simulink model "BaseEngineController_LS_128"  (Simulink 7.7)
settings: Solver=FixedStepDiscrete  StartTime=0.0  StopTime=10.0  RelTol=1e-3
PreLoadFcn:
  | try, eval([bdroot '_setup']); catch, eval('model_setup', ''); end
InitFcn:
  | try, eval([bdroot '_setup']); catch, eval('model_setup', ''); end
undefined symbols (not defined in the file): ECU565, High, motohawk_build_version, motohawk_trunc_name, motohawk_vardec_config_group, motohawk_vardec_path, True
libraries: MotoHawk_lib x1418, motohawk_control_primitives_lib x183, motohawk_engine_lib x32, simulink x21, motohawk_annotations_lib x9, AutoDoc_lib x8, simulink_extras x4, motohawk_ccp_examples_lib x1, motohawk_control_primitives_motoshare_lib x1
(part 2 of 27)

== system BaseEngineController_LS_128/Foreground/Control/ActuatorCharacterization ==
  Control : Inport
  Sensors : Inport  Port=2
  Diagnsotics : Inport  Port=3
  Bus Creator1 : BusCreator  Inputs=8
  Bus Creator3 : BusCreator
  Bus Selector1 : BusSelector  OutputSignals=AirCalcs.Baro,Raw.LinearSensors.MAP_Angular,RawIndexes.SysVolt09Idx,Raw.RPM,Raw.LinearSensors.FuelPres
  Bus Selector3 : BusSelector  OutputSignals=RawProcessed.TPS
  Bus Selector4 : BusSelector  OutputSignals=Throttle
  Bus Selector5 : BusSelector  OutputSignals=SparkAdv,SparkEnergy,FPC
  CompareTo : motohawk_control_primitives_lib/CompareTo  SystemSampleTime=-1  op===  val=0
  Electronic Throttle Controller : Subsystem  TreatAsAtomicUnit=on
      mask Display:
      | patch([0 0 1 1], [0 0.075 0.075 0], [230/255 0/255 0/255])
      | patch([0 0 1 1], [0.025 0.05 0.05 0.025], [150/255 0/255 0/255])
      | patch([0 0 1 1], [0 0.025 0.025 0], [0/255 0/255 0/255])
      | 
      | disp('Electronic Throttle');
  Injector Characterization : Subsystem  Description=|
      | /* Name: InjGain Unit:ms/mg ClassID:VAR StorageID:FLASH Access:RW4+RW3+NA2+NA1 TypeID:UINT2 Gain:0.0001       
      |    Min:0.0000 Max:6.5500 Format:5.4 UpdateID:REMOTE Group:"Actuators | Injectors | Config" Help:"Gain valued "
      |    "used in the linear transformation of FPC to mechanical pulsewidth." VardecSig:6C */                       
      |                                                                                                               
      | /* Name: InjOfst Unit:ms ClassID:VAR StorageID:FLASH Access:RW4+RW3+NA2+NA1 TypeID:SINT2 Gain:0.0001          
      |    Min:-3.2768 Max:3.2767 Format:5.4 UpdateID:REMOTE Group:"Actuators | Injectors | Config" Help:"Offset "    
      |    "valued used in the linear transformation of FPC to mechanical pulsewidth." VardecSig:6C */                
      |                                                                                                               
      | /* Name: SysVolt10IdxArr Unit:volt ClassID:ORDARR StorageID:FLASH Access:RW4+RW3+NA2+NA1 TypeID:UINT1         
      |    Gain:0.1 Min:0.00 Max:25.50 Format:4.2 UpdateID:REMOTE OrdLen:10 Group:"Global Index Arrays | Voltage"     
      |    Help:"Ten breakpoint system voltage index array." VardecSig:6C */                                          
      |                                                                                                               
      | /* Name: InjTurnOnTbl Unit:ms ClassID:TBL StorageID:FLASH Access:RW4+RW3+NA2+NA1 TypeID:UINT2 Gain:0.001      
      |    Min:0.0000 Max:65.5350 Format:5.4 UpdateID:REMOTE OrdArr:SysVolt10IdxArr Group:"Actuators | Injectors"     
      |    Help:"Injector turn on time as a function of system voltage." VardecSig:6C */                              
      |                                                                                                               
      | /* Name: InjDeltaPress10IdxArr Unit:kPa ClassID:ORDARR StorageID:FLASH Access:RW4+RW3+NA2+NA1 TypeID:UINT2    
      |    Gain:0.1 Min:0.0 Max:6553.0 Format:5.1 UpdateID:REMOTE OrdLen:10 Group:"Actuators | Injectors" Help:"Ten " 
      |    "breakpoint fuel delta pressure index array." VardecSig:6C */                                              
      |                                                                                                               
      | /* Name: FueldPCompTbl Unit:kPa ClassID:TBL StorageID:FLASH Access:RW4+RW3+NA2+NA1 TypeID:UINT2 Gain:0.1      
      |    Min:0.0 Max:6553.0 Format:5.1 UpdateID:REMOTE OrdArr:InjDeltaPress10IdxArr Group:"Actuators | Injectors"   
      |    Help:"Injector delta pressure compensation table." VardecSig:6C */                                         
      |                                                                                                               
      | /* Name: InjTurnOffTbl Unit:ms ClassID:TBL StorageID:FLASH Access:RW4+RW3+NA2+NA1 TypeID:UINT2                
      |    Gain:0.01 Min:0.00 Max:655.00 Format:5.2 UpdateID:REMOTE OrdArr:InjDeltaPress10IdxArr Group:"Actuators | " 
      |    "Injectors" Help:"Injector turn off time table." VardecSig:6C */                                           
      |                                                                                                               
      | /* Name: InjMPW Unit:ms ClassID:VAR StorageID:RAM Access:RO4+RO3+NA2+NA1 TypeID:UINT2 Gain:0.01 Min:0.00      
      |    Max:655.35 Format:5.2 UpdateID:BACKGND Group:"Actuators | Injectors" Help:"Injector mechanical pulse "     
      |    "width." VardecSig:6C */                                                                                   
      |                                                                                                               
      | /* Name: InjEPW Unit:ms ClassID:VAR StorageID:RAM Access:RO4+RO3+NA2+NA1 TypeID:UINT2 Gain:0.01 Min:0.00      
      |    Max:655.35 Format:5.2 UpdateID:BACKGND Group:"Actuators | Injectors" Help:"Injector electrical pulse "     
      |    "width." VardecSig:6C */                                                                                   
      |                                                                                                               
      | /* Name: InjDeltaPress Unit:kPa ClassID:VAR StorageID:RAM Access:RO4+RO3+NA2+NA1 TypeID:UINT2 Gain:0.01       
      |    Min:0.00 Max:655.35 Format:5.2 UpdateID:BACKGND Group:"Actuators | Injectors" Help:"Delta pressure across "
      |    "the injector." VardecSig:6C */                                                                            
      | /* Name: FuelFlowCompMap Unit:mult ClassID:MAP StorageID:RAM Access:RO4+RO3+NA2+NA1 TypeID:UINT2              
      |    Gain:0.0001 Min:0.0000 Max:2.0000 Format:5.4 UpdateID:BACKGND XOrdArr:IndTorque10IdxArr YOrdArr:RPM10IdxArr
      |    Group:"Actuators | Injectors" Help:"Correction for injector fuel flow differences between injector test "  
      |    "bench and engine operating in the conditions. This map should only be calibrated after volumetric "       
      |    "efficiency has been calibrated to a reference airflow measurement device." VardecSig:6C */
      mask Description: Injector characterization block.
      mask Help: Converts the calculated fuel charge mass (FPC) value to the required electrical pulsewidth. Requires gain, offset, turn-on time vs. voltage, turn-off time vs. injector delta pressure and delta pressure pulsewidth compensation. A choice of five different injector delta pressure calculation methods are offered.
      mask Display:
      | patch([0 0 1 1], [0 0.075 0.075 0], [230/255 0/255 0/255])
      | patch([0 0 1 1], [0.025 0.05 0.05 0.025], [150/255 0/255 0/255])
      | patch([0 0 1 1], [0 0.025 0.025 0], [0/255 0/255 0/255])
      | 
      | disp('INJECTOR\nCHRZN.\n(High Z Only)')
  SequenceCutPattern : Subsystem
      mask Display:
      | patch([0 0 1 1], [0 0.075 0.075 0], [230/255 0/255 0/255])
      | patch([0 0 1 1], [0.025 0.05 0.05 0.025], [150/255 0/255 0/255])
      | patch([0 0 1 1], [0 0.025 0.025 0], [0/255 0/255 0/255])
      | 
      | disp('REV LIMITER\nACTION\n8 CYLINDER')
  Spark Advance to Start Angle : Subsystem  Description=|  TreatAsAtomicUnit=on
      | /* Name: CoilDrvrDlyTime Unit:us ClassID:VAR StorageID:FLASH Access:RW4+RW3+NA2+NA1 TypeID:UINT2 Gain:0.1       
      |    Min:0.00 Max:6553.50 Format:6.2 UpdateID:REMOTE Group:"Actuators | Coils" Help:"Coil driver delay time "     
      |    "between initiation of the EST signal and the initiation of coil dwell." VardecSig:6C */                     
      |                                                                                                                 
      | /* Name: SysVolt10IdxArr Unit:volt ClassID:VAR StorageID:FLASH Access:RW4+RW3+NA2+NA1 TypeID:UINT1 Gain:0.1     
      |    Min:0.00 Max:25.50 Format:4.2 UpdateID:REMOTE Group:"Global Index Arrays | Voltage" Help:"Ten breakpoint "   
      |    "system voltage index array." VardecSig:6C */                                                                
      |                                                                                                                 
      | /* Name: SpkEnergy10IdxArr Unit:volt ClassID:VAR StorageID:FLASH Access:RW4+RW3+NA2+NA1 TypeID:UINT1            
      |    Gain:0.1 Min:0.00 Max:25.50 Format:4.2 UpdateID:REMOTE Group:"Actuators | Coils" Help:"Ten breakpoint spark "
      |    "energy index array." VardecSig:6C */                                                                        
      |                                                                                                                 
      | /* Name: CoilDwellMap Unit:ms ClassID:MAP StorageID:FLASH Access:RW4+RW3+NA2+NA1 TypeID:UINT2 Gain:0.01         
      |    Min:0.00 Max:655.35 Format:4.2 UpdateID:REMOTE XOrdArr:SpkEnergy10IdxArr YOrdArr:SysVolt10IdxArr             
      |    Group:"Actuators | Coils" Help:"Required coil dwell map as a function of system voltage and spark energy."   
      |    VardecSig:6C */
      mask Type: Stop Angle to Start Angle
      mask Description: Stop Angle to Start Angle calculation.  Subtracts the duration of a Pulse Width in the angle domain from a given Stop Angle.
      mask Display:
      | patch([0 0 1 1], [0 0.075 0.075 0], [230/255 0/255 0/255])
      | patch([0 0 1 1], [0.025 0.05 0.05 0.025], [150/255 0/255 0/255])
      | patch([0 0 1 1], [0 0.025 0.025 0], [0/255 0/255 0/255])
  Spark Coil Characterization : Subsystem  Description=|  TreatAsAtomicUnit=on
      | /* Name: CoilDrvrDlyTime Unit:us ClassID:VAR StorageID:FLASH Access:RW4+RW3+NA2+NA1 TypeID:UINT2 Gain:0.1       
      |    Min:0.00 Max:6553.50 Format:6.2 UpdateID:REMOTE Group:"Actuators | Coils" Help:"Coil driver delay time "     
      |    "between initiation of the EST signal and the initiation of coil dwell." VardecSig:6C */                     
      |                                                                                                                 
      | /* Name: SysVolt10IdxArr Unit:volt ClassID:VAR StorageID:FLASH Access:RW4+RW3+NA2+NA1 TypeID:UINT1 Gain:0.1     
      |    Min:0.00 Max:25.50 Format:4.2 UpdateID:REMOTE Group:"Global Index Arrays | Voltage" Help:"Ten breakpoint "   
      |    "system voltage index array." VardecSig:6C */                                                                
      |                                                                                                                 
      | /* Name: SpkEnergy10IdxArr Unit:volt ClassID:VAR StorageID:FLASH Access:RW4+RW3+NA2+NA1 TypeID:UINT1            
      |    Gain:0.1 Min:0.00 Max:25.50 Format:4.2 UpdateID:REMOTE Group:"Actuators | Coils" Help:"Ten breakpoint spark "
      |    "energy index array." VardecSig:6C */                                                                        
      |                                                                                                                 
      | /* Name: CoilDwellMap Unit:ms ClassID:MAP StorageID:FLASH Access:RW4+RW3+NA2+NA1 TypeID:UINT2 Gain:0.01         
      |    Min:0.00 Max:655.35 Format:4.2 UpdateID:REMOTE XOrdArr:SpkEnergy10IdxArr YOrdArr:SysVolt10IdxArr             
      |    Group:"Actuators | Coils" Help:"Required coil dwell map as a function of system voltage and spark energy."   
      |    VardecSig:6C */
      mask Description: Coil characterization block.
      mask Help: Given the desired spark energy and system voltage, this block determines the required coil dwell period. Requires calibration of the dwell map and the delay time.
      mask Display:
      | patch([0 0 1 1], [0 0.075 0.075 0], [230/255 0/255 0/255])
      | patch([0 0 1 1], [0.025 0.05 0.05 0.025], [150/255 0/255 0/255])
      | patch([0 0 1 1], [0 0.025 0.025 0], [0/255 0/255 0/255])
      | 
      | disp('COIL\nCHRZN.')
  motohawk_data_read : MotoHawk_lib/Data Storage Blocks/motohawk_data_read  source=Lookup By Name  structure=Scalar  operation=Read scalar from location by index  sz_vec=4  sz_row=2  sz_col=3  typ=boolean  nam='AirControlSource'  checkNull=on  struct_inst_name='Struct1'  struct_nam='MyStruct'
  motohawk_trigger : MotoHawk_lib/Trigger Blocks/motohawk_trigger  Tag=Trigger  trigger=FGND_5XRTI_PERIODIC  function_name=Trigger_FGND_5XRTI_PERIODIC_1093p0005  priority_order=1  inherited=on  run_disabled=off  override_app_monitor=off  target=ECU565_128
  motohawk_trigger1 : MotoHawk_lib/Trigger Blocks/motohawk_trigger  Tag=Trigger  trigger=FGND_5XRTI_PERIODIC  function_name=Trigger_FGND_5XRTI_PERIODIC_1094p0005  priority_order=1  inherited=on  run_disabled=off  override_app_monitor=off  target=ECU565_128
  Actuators : Outport
  wires:
  Sensors/1 -> Bus Selector1/1, Bus Creator3/3, Bus Selector3/1  "Sensors"
  Bus Selector3/1 -> Electronic Throttle Controller/1(TPS)  "<TPS>"
  Electronic Throttle Controller/1(ETC) -> Bus Creator1/5  "ETC"
  Bus Selector4/1 -> Electronic Throttle Controller/2(ETCReq)  "<Throttle>"
  Control/1 -> Bus Selector5/1, Bus Creator3/2, Bus Selector4/1  "Controller"
  Bus Selector1/3 -> Injector Characterization/4(SysVolt09Idx), Spark Coil Characterization/2(SysVolt09Idx)  "<SysVolt09Idx>"
  Bus Selector1/4 -> Spark Advance to Start Angle/2(RPM), Injector Characterization/5(RPM)  "<RPM>"
  Spark Advance to Start Angle/1(Start Angle [degCA]) -> Bus Creator1/3  "SparkStartAngle"
  Spark Coil Characterization/1(SparkDwell [ms]) -> Spark Advance to Start Angle/3(PulseWidth [ms])  "SparkDwell"
  Bus Selector1/2 -> Injector Characterization/3(MAP [kPa])  "<MAP_Angular>"
  Bus Selector1/1 -> Injector Characterization/2(BaroPress [kPa])  "<Baro>"
  Injector Characterization/1(MPW [ms]) -> Bus Creator1/1  "InjMPW"
  Bus Selector5/1 -> Spark Advance to Start Angle/1(Stop Angle [degCA])  "<SparkAdv>"
  Bus Selector5/2 -> Spark Coil Characterization/1(SparkEnergy [mJ])  "<SparkEnergy>"
  Spark Coil Characterization/2(SparkEnable [bool]) -> Bus Creator1/4  "SparkEnable"
  Injector Characterization/2(EPWOffset [ms]) -> Bus Creator1/2  "InjEPWOffset"
  SequenceCutPattern/1(Spark) -> Bus Creator1/6  "SparkCutSeq"
  SequenceCutPattern/2(Fuel) -> Bus Creator1/7  "FuelCutSeq"
  Bus Creator3/1 -> Actuators/1  "Engine"
  Bus Creator1/1 -> Bus Creator3/4  "ActuatorCharacterization"
  Diagnsotics/1 -> Bus Creator3/1  "Diagnsotics"
  motohawk_trigger/1 -> Spark Advance to Start Angle/Trigger
  motohawk_trigger1/1 -> Spark Coil Characterization/Trigger
  motohawk_data_read/1 -> CompareTo/1
  CompareTo/1 -> Electronic Throttle Controller/Enable
  Electronic Throttle Controller/2(ETC_TestActive) -> Bus Creator1/8  "ETC_TestActive"
  Bus Selector1/5 -> Injector Characterization/6(FuelPress [kPa])  "<FuelPres>"
  Bus Selector5/3 -> Injector Characterization/1(FPC [mg])  "<FPC>"

== system BaseEngineController_LS_128/Foreground/Control/Controller ==
  Sensors : Inport
  Bus Selector : BusSelector  OutputSignals=RawProcessed.EngineState
  Crank : Subsystem  TreatAsAtomicUnit=on
      mask Display: disp('CRANK STATE\nALGORITHM');
  Crank State : motohawk_control_primitives_lib/CompareTo  SystemSampleTime=-1  op===  val=2
  Merge : Subsystem
  Run : Subsystem  TreatAsAtomicUnit=on
      mask Display: disp('RUN STATE\nALGORITHM');
  Run State : motohawk_control_primitives_lib/CompareTo  SystemSampleTime=-1  op===  val=3
  Stall : Subsystem  TreatAsAtomicUnit=on
      mask Display: disp('STALL STATE\nALGORITHM');
  Stall State : motohawk_control_primitives_lib/CompareTo  SystemSampleTime=-1  op===  val=1
  Actuators : Outport
  DesEquivRatio : Outport  Port=2
  wires:
  Sensors/1 -> Bus Selector/1, Crank/1(Inputs), Run/1(Inputs), Stall/1(Inputs)
  Stall State/1 -> Stall/Enable
  Crank State/1 -> Crank/Enable
  Run State/1 -> Run/Enable
  Stall/1(Actuators) -> Merge/1(Stall)
  Run/1(Actuators) -> Merge/3(Run)
  Crank/1(Actuators) -> Merge/2(Crank)
  Bus Selector/1 -> Stall State/1, Run State/1, Crank State/1  "<EngineState>"
  Merge/1(Actuators) -> Actuators/1
  Run/2(DesEquivRatio) -> DesEquivRatio/1

== system BaseEngineController_LS_128/Foreground/Control/Diagnostics ==
  Control : Inport
  Sensors : Inport  Port=2
  DesEquivRatio : Inport  Port=3
  Trigger : TriggerPort  TriggerType=function-call
  AC Fault : Subsystem
  AirFlow : Subsystem
  Boost Fault : Subsystem
  Bus Creator1 : BusCreator
  Bus Selector : BusSelector  OutputSignals=Raw.RPMInst
  Digital Sensors : Subsystem
  Engine Overheat Fault Logic : Subsystem
  Fuel Economy : Subsystem
  Lean Protect : Subsystem
  Low Oil Pressure Fault Logic : Subsystem
  Low Voltage : Subsystem
  MAP Fault Logic : Subsystem
  MISFIRE : Subsystem
  O2 Smart Sensor : Subsystem
  Overspeed Protection : Subsystem  AncestorBlock=motohawk_engine_lib/Overspeed Protection
      mask Description:
      | Block allows for three levels of overspeed rev limits, and will set three fault accordingly.
      | 
      | Soft Overspeed, Medium Overspeed, and Hard Overspeed.
      mask Display:
      | patch([0 0 1 1], 0.5*[0 0.075 0.075 0], [230/255 0/255 0/255])
      | patch([0 0 1 1], 0.5*[0.025 0.05 0.05 0.025], [150/255 0/255 0/255])
      | patch([0 0 1 1], 0.5*[0 0.025 0.025 0], [0/255 0/255 0/255])
      | 
      | disp('RPM LIMITER');
  Terminator2 : Terminator
  Wrong Fuel Pressure Fault Logic : Subsystem
  Diagnostics : Outport
  wires:
  Bus Creator1/1 -> Diagnostics/1  "Diagnostics"
  Sensors/1 -> Bus Selector/1, Engine Overheat Fault Logic/1(Sensors), MAP Fault Logic/1(Sensors), Low Oil Pressure Fault Logic/1(Sensors), Fuel Economy/1(Sensors), Wrong Fuel Pressure Fault Logic/1(Sensors), Boost Fault/1(Sensors), AC Fault/1(Sensors), Lean Protect/1(Sensors), Low Voltage/1(Sensors), Digital Sensors/1(Sensors), O2 Smart Sensor/1(Sensors), MISFIRE/1(Sensors), AirFlow/1(Sensors)
  Control/1 -> Terminator2/1, Fuel Economy/2(Controller), Boost Fault/2(Controller), AC Fault/2(Controller)  "Control"
  Bus Selector/1 -> Overspeed Protection/1(RPM)  "<RPMInst>"
  Fuel Economy/1(FuelEconomy_instantaneous) -> Bus Creator1/3  "FuelEconomy_instantaneous"
  Fuel Economy/2(FuelEconomy_filtered) -> Bus Creator1/4  "FuelEconomy_filtered"
  Low Oil Pressure Fault Logic/1(LowOilPres) -> Bus Creator1/2  "LowOilPres"
  Engine Overheat Fault Logic/1(Overheat_Warning) -> Bus Creator1/1  "Overheat_Warning"
  DesEquivRatio/1 -> O2 Smart Sensor/2(DesEquivRatio)

== system BaseEngineController_LS_128/Foreground/Control/VirtualSensors ==
  Raw : Inport
  AirCalcs : Subsystem
  Bus Creator : BusCreator  Inputs=7
  FuelLevel : Subsystem
  LoadBasedCalcs : Subsystem
  Raw Indexes : Subsystem
  RawProcessed : Subsystem
  Virtual Indexes : Subsystem
  Sensors : Outport
  wires:
  Raw/1 -> RawProcessed/1(Raw), Raw Indexes/1(Raw), AirCalcs/2(Raw), LoadBasedCalcs/1(RAW), FuelLevel/1(Sensors), Bus Creator/1  "Raw"
  Bus Creator/1 -> Sensors/1  "SynthSensors"
  RawProcessed/1(RawProcessed) -> Bus Creator/2, AirCalcs/4(RawProcessed), Virtual Indexes/2(RawProcessed), FuelLevel/2(Raw Processed), Raw Indexes/2(RawProcessed)  "RawProcessed"
  Raw Indexes/1(RawIndexes) -> Bus Creator/3, AirCalcs/1(RawIndexes), RawProcessed/2(Indexes)  "RawIndexes"
  AirCalcs/1(AirCalcs) -> Bus Creator/4, Virtual Indexes/1(AirCalcs)  "AirCalcs"
  LoadBasedCalcs/1(SSEng) -> Bus Creator/5, AirCalcs/3(SSEngOpr)  "SSEng"
  Virtual Indexes/1(VirtualIndexes) -> Bus Creator/6  "VirtualIndexes"
  FuelLevel/1(Fuel Lvl Final) -> Bus Creator/7  "FuelLvl_Fin"

== system BaseEngineController_LS_128/Foreground/Inputs/CAN ==
  AEM GPS : Subsystem
  AEM X Lambda : Subsystem
  Bus Creator1 : BusCreator
  SensorBus : Outport
  wires:
  Bus Creator1/1 -> SensorBus/1  "CAN"
  AEM X Lambda/1(O2_BankA) -> Bus Creator1/1  "O2_BankA"
  AEM GPS/1(GPS_BUS) -> Bus Creator1/4  "GPS_BUS"
  AEM X Lambda/3(O2_BUS) -> Bus Creator1/3  "O2_BUS"
  AEM X Lambda/2(O2_BankB) -> Bus Creator1/2  "O2_BankB"

== system BaseEngineController_LS_128/Foreground/Inputs/Digital ==
  "ACSw " : motohawk_engine_lib/Analog Switch  SystemSampleTime=-1  nam='ACSw'  prefix='ACSw'  switchpoint=500  polarity=High-True  parent_group=motohawk_vardec_path(gcb)
  Bus Creator : BusCreator  Inputs=6
  ClutchSw : motohawk_engine_lib/Analog Switch  SystemSampleTime=-1  nam='ClutchSw'  prefix='ClutchSw'  switchpoint=500  polarity=High-True  parent_group=motohawk_vardec_path(gcb)
  Data Type Conversion : DataTypeConversion
  Data Type Conversion1 : DataTypeConversion
  ESTOP : motohawk_engine_lib/Analog Switch1  SystemSampleTime=-1  nam='ESTOP'  prefix='ESTOP'  polarity=High-True  parent_group=motohawk_vardec_path(gcb)
  Gain : Gain  Gain=.01
  Gain1 : Gain  Gain=.01
  MAF_Sensor : motohawk_engine_lib/Non-Linear Sensor Characterization (tbl)  SystemSampleTime=-1  nam='MAF'  prefix='MAF'  units='g/s'  inputunits='Hz'  parent_group=motohawk_vardec_path(gcb)  tblsize=13  samp_time=-1
  "Scramble " : Subsystem  AncestorBlock=motohawk_engine_lib/Analog Switch  mask{nam='Scramble', prefix='Scramble', switchpoint=500, polarity=High-True, parent_group=motohawk_vardec_path(gcb)}
      mask prompts: nam "Name"; switchpoint "Switch Point (ADC)"; parent_group "MotoTune Group"
      mask init:
      | lbl = ['Analog Switch: ' nam ' [bool]'];
      | group = [parent_group ' | ' nam];
      mask StyleString: edit,edit,edit,popup(High-True|Low-True),edit
      mask Display:
      | patch([0 0 1 1], [0 0.075 0.075 0], [230/255 0/255 0/255])
      | patch([0 0 1 1], [0.025 0.05 0.05 0.025], [150/255 0/255 0/255])
      | patch([0 0 1 1], [0 0.025 0.025 0], [0/255 0/255 0/255])
      | 
      | disp(lbl);
  Terminator{1..4} (4 alike) : Terminator
  VSPD : motohawk_engine_lib/Non-Linear Sensor Characterization (tbl)  SystemSampleTime=-1  nam='VSPD'  prefix='VSPD'  units='MPH'  inputunits='Hz'  parent_group=motohawk_vardec_path(gcb)  tblsize=5  samp_time=-1
  VSPD_Filt : Subsystem
  motohawk_ain1 : MotoHawk_lib/Analog I//O Blocks/motohawk_ain  res_name=[]  text_resource=AN15M  code_resource=RES_ECUP  val_resource=-1  target=ECU565-128  resource_enum_str=(None)=-1,ECUP=53,DRVP=54,XDRP=55,AN1M=56,AN2M=57,AN3M=58,AN4M=59,AN5M=60,AN6M=61,AN7M=62,AN8M=63,AN9M=64,AN10M=65,AN11M=66,AN12M=67,AN13M=68,AN14M=69,AN15M=70,AN16M=71,AN17M=72,AN18M=73,AN19M=74,AN20M=75,AN21M=76,AN22M=77,AN23M=78,AN24M=79,AN25M=80,AN26M=81,AN27M=82,AN28M=83,AN29M=84,AN30M=85,AN31M=86,AN32M=87,AN33M=88,AN34M=89,O2A=90,O2B=91,XDRP_B=92,REF_14V=143  altref=5V Reference  typ=uint16  num_adc_bits=10  use_stat=off  use_vardec=on  nam='ClutchSw_Pin'  read_level=1  write_level=1  group='System | I/O Pins | Inputs Config'
  motohawk_ain5 : MotoHawk_lib/Analog I//O Blocks/motohawk_ain  res_name=[]  text_resource=AN15M  code_resource=RES_ECUP  val_resource=-1  target=ECU565-128  resource_enum_str=(None)=-1,ECUP=53,DRVP=54,XDRP=55,AN1M=56,AN2M=57,AN3M=58,AN4M=59,AN5M=60,AN6M=61,AN7M=62,AN8M=63,AN9M=64,AN10M=65,AN11M=66,AN12M=67,AN13M=68,AN14M=69,AN15M=70,AN16M=71,AN17M=72,AN18M=73,AN19M=74,AN20M=75,AN21M=76,AN22M=77,AN23M=78,AN24M=79,AN25M=80,AN26M=81,AN27M=82,AN28M=83,AN29M=84,AN30M=85,AN31M=86,AN32M=87,AN33M=88,AN34M=89,O2A=90,O2B=91,XDRP_B=92,REF_14V=143  altref=5V Reference  typ=uint16  num_adc_bits=10  use_stat=off  use_vardec=on  nam='ACSwPin'  read_level=1  write_level=1  group='System | I/O Pins | Inputs Config'
  motohawk_ain6 : MotoHawk_lib/Analog I//O Blocks/motohawk_ain  res_name=[]  text_resource=AN19M  code_resource=RES_ECUP  val_resource=-1  target=ECU565-128  resource_enum_str=(None)=-1,ECUP=53,DRVP=54,XDRP=55,AN1M=56,AN2M=57,AN3M=58,AN4M=59,AN5M=60,AN6M=61,AN7M=62,AN8M=63,AN9M=64,AN10M=65,AN11M=66,AN12M=67,AN13M=68,AN14M=69,AN15M=70,AN16M=71,AN17M=72,AN18M=73,AN19M=74,AN20M=75,AN21M=76,AN22M=77,AN23M=78,AN24M=79,AN25M=80,AN26M=81,AN27M=82,AN28M=83,AN29M=84,AN30M=85,AN31M=86,AN32M=87,AN33M=88,AN34M=89,O2A=90,O2B=91,XDRP_B=92,REF_14V=143  altref=5V Reference  typ=uint16  num_adc_bits=10  use_stat=off  use_vardec=on  nam='ScramblePin'  read_level=1  write_level=1  group='System | I/O Pins | Inputs Config'
  motohawk_callout1 : motohawk_annotations_lib/motohawk_callout1  BlockType_='Mototron_harea'  desc='\fontsize{12}Read from H/W'  edit_text=Compute the mean forward body acceleration.Worry about rounding.  edit_as=255
  motohawk_callout2 : motohawk_annotations_lib/motohawk_callout1  BlockType_='Mototron_harea'  desc='\fontsize{12}Convert to Engineering Units'  edit_text=Compute the mean forward body acceleration.Worry about rounding.  edit_as=255
  motohawk_callout3 : motohawk_annotations_lib/motohawk_callout1  BlockType_='Mototron_harea'  desc='\fontsize{12}Create a Bus of Sensors'  edit_text=Compute the mean forward body acceleration.Worry about rounding.  edit_as=255
  motohawk_din : MotoHawk_lib/Digital I//O Blocks/motohawk_din  resource_name=[]  text_resource=O2A  code_resource=NONE  val_resource=-1  target=ECU565-128  resource_enum_str=(None)=-1,AN1M=56,AN2M=57,AN3M=58,AN4M=59,AN5M=60,AN6M=61,AN7M=62,AN8M=63,AN9M=64,AN10M=65,AN11M=66,AN12M=67,AN13M=68,AN14M=69,AN15M=70,AN16M=71,AN17M=72,AN18M=73,AN19M=74,AN20M=75,AN21M=76,AN22M=77,AN23M=78,AN24M=79,AN25M=80,AN26M=81,AN27M=82,AN28M=83,AN29M=84,AN30M=85,AN31M=86,AN32M=87,AN33M=88,AN34M=89,O2A=90,O2B=91,DG1M=93,DG2M=94,DG3M=95,DG4M=96,DG5M=102,DG6M=103,DG7M=104,SPD1=105,SPD2=106,DG8M=111  pullup=None  use_stat=off  use_vardec=on  nam='ESTOPPin'  read_level=1  write_level=1  group='System | I/O Pins | Inputs Config'
  motohawk_frequency_in1 : MotoHawk_lib/Advanced Digital I//O/motohawk_frequency_in  res_name=[]  text_resource=DG4M  code_resource=RES_DG1M  val_resource=-1  target=ECU565-128  resource_enum_str=(None)=-1,DG1M=93,DG2M=94,DG3M=95,DG4M=96,DG5M=102,DG6M=103,DG7M=104,SPD1=105,SPD2=106,DG8M=111  ipwm=Perform Duty Cycle Measument  itrig=off  Nmax=8  edge=Falling Edge  alias=Disabled  min_freq=10  sig=Digital Input  use_vardec=on  nam='VSPD_Pin'  read_level=1  write_level=1  group='System | I/O Pins | Inputs Config'  cal_group='System | I/O Pins | Frequency In Config'
  motohawk_frequency_in2 : MotoHawk_lib/Advanced Digital I//O/motohawk_frequency_in  res_name=[]  text_resource=DG2M  code_resource=RES_DG1M  val_resource=-1  target=ECU565-128  resource_enum_str=(None)=-1,DG1M=93,DG2M=94,DG3M=95,DG4M=96,DG5M=102,DG6M=103,DG7M=104,SPD1=105,SPD2=106,DG8M=111  ipwm=Perform Duty Cycle Measument  itrig=off  Nmax=8  edge=Falling Edge  alias=Disabled  min_freq=10  sig=Digital Input  use_vardec=on  nam='MAF_Pin'  read_level=1  write_level=1  group='System | I/O Pins | Inputs Config'  cal_group='System | I/O Pins | Frequency In Config'
  SensorBus : Outport
  wires:
  Bus Creator/1 -> SensorBus/1  "Digital"
  motohawk_frequency_in2/1 -> Data Type Conversion/1
  MAF_Sensor/2 -> Terminator4/1
  Data Type Conversion/1 -> Gain/1
  Gain/1 -> MAF_Sensor/1
  motohawk_frequency_in2/2 -> Terminator1/1
  motohawk_ain5/1 -> "ACSw "/1
  motohawk_ain6/1 -> "Scramble "/1(ADC)
  motohawk_din/1 -> ESTOP/1
  MAF_Sensor/1 -> Bus Creator/1  "MAF"
  ESTOP/1 -> Bus Creator/2  "ESTOP"
  motohawk_frequency_in1/1 -> Data Type Conversion1/1
  Data Type Conversion1/1 -> Gain1/1
  Gain1/1 -> VSPD/1
  motohawk_frequency_in1/2 -> Terminator2/1
  VSPD/2 -> Terminator3/1
  motohawk_ain1/1 -> ClutchSw/1
  VSPD/1 -> VSPD_Filt/1(In1)  "VSPD"
  "ACSw "/1 -> Bus Creator/3  "ACSw"
  "Scramble "/1(DiscOut) -> Bus Creator/4  "Scramble"
  VSPD_Filt/1(Out1) -> Bus Creator/5  "VSPD"
  ClutchSw/1 -> Bus Creator/6  "ClutchSw"

== system BaseEngineController_LS_128/Foreground/Inputs/EngineSpeed ==
  note: Set PseudoRPM from MotoTune
      | to a non-zero value to cause
      | simulated RPM
  Constant : Constant  Value=0  OutDataTypeStr=Inherit: Inherit via back propagation
  Data Type Conversion : DataTypeConversion  SaturateOnIntegerOverflow=on  RndMeth=Zero
  Data Type Conversion1 : DataTypeConversion  OutDataTypeStr=double  SaturateOnIntegerOverflow=on  RndMeth=Zero
  Data Type Conversion3 : DataTypeConversion  RndMeth=Zero
  Encoder Diagnostics : Subsystem
  First Order Low Pass (Tunable)1 : motohawk_control_primitives_lib/First Order Low Pass (Tunable)  SystemSampleTime=-1  nam='RPMFiltConst'  samp_time=-1  group=motohawk_vardec_path(gcb)
  Gain : Gain  Gain=16  SaturateOnIntegerOverflow=on  OutDataTypeStr=Inherit: Same as input  ParamDataTypeStr=Inherit: Same as input
  Relational Operator : RelationalOperator  Operator=~=  ZeroCross=off  InputSameDT=on
  motohawk_calibration : MotoHawk_lib/Calibration & Probing Blocks/motohawk_calibration  nam='PseudoRPM'  val=0  storage=Calibration  show_more=on  name_source=Use Parameter  data_type=Inherit via back propagation  read_level=1  write_level=1  ovr_cals=on  view_as=Number  enum_struct={'Disabled', 'Enabled'}  vector_style=Wide Row  use_help_units=off  help=''  units=''  use_header_enum=off  row_header_enum={}  col_header_enum={}  use_min_max=off  min_val=-inf  max_val=inf  use_precision=off  precision=''  gain=1  offset=0  exp=1  use_mototune_group=on  mototune_group=motohawk_vardec_path(gcb)
  motohawk_calibration1 : MotoHawk_lib/Calibration & Probing Blocks/motohawk_calibration  nam='EngineToEncoderOffset'  val=0  storage=Calibration  show_more=on  name_source=Use Parameter  data_type=Inherit from 'Default Value'  read_level=1  write_level=1  ovr_cals=on  view_as=Number  enum_struct={'Disabled', 'Enabled'}  vector_style=Wide Row  use_help_units=on  help=''  units=''  use_header_enum=off  row_header_enum={}  col_header_enum={}  use_min_max=off  min_val=-inf  max_val=inf  use_precision=off  precision=''  gain=1  offset=0  exp=1  use_mototune_group=on  mototune_group=motohawk_vardec_path(gcb)
  motohawk_encoder_average_rpm : MotoHawk_lib/Encoder Blocks/motohawk_encoder_average_rpm
  motohawk_encoder_def : MotoHawk_lib/Encoder Blocks/motohawk_encoder_def  encoder_type=GM 24Xe - 4-Stroke - Half-Moon CAM  interface=Digital Crank - Digital Cam  sync=Rising Edge  crnkpullup=Strong Pullup  camsync=Rising Edge  campullup=Strong Pullup  angle_offset=27  sec_tdcoffset=-34.3  cam_delay=0  teeth_after_cam=-1  ignore_teeth=6  ignore_delay=100  angles=[0 270 630 540 450 360 180 90]  cnk_align_with_cam=off  adaptive_vr_cnk=off  adaptive_vr_cam=on  cal_cylinders=on  max_cylinders=8  num_cylinders=8  read_level=1  write_level=1  ovr_cals=on  group=motohawk_vardec_path(gcb)
  motohawk_encoder_fault : MotoHawk_lib/Encoder Blocks/motohawk_encoder_fault
  motohawk_encoder_instant_rpm : MotoHawk_lib/Encoder Blocks/motohawk_encoder_instant_rpm
  motohawk_encoder_offset : MotoHawk_lib/Encoder Blocks/motohawk_encoder_offset
  motohawk_encoder_pseudo : MotoHawk_lib/Encoder Blocks/motohawk_encoder_pseudo
  motohawk_encoder_state : MotoHawk_lib/Encoder Blocks/motohawk_encoder_state
  motohawk_probe : MotoHawk_lib/Calibration & Probing Blocks/motohawk_probe  nam='RPMInst'  show_more=on  name_source=Use Parameter  read_level=1  view_as=Number  enum_struct={'Disabled', 'Enabled'}  vector_style=Wide Row  use_help_units=off  help=''  units=''  use_header_enum=off  row_header_enum={}  col_header_enum={}  use_precision=off  precision=''  gain=1  offset=0  exp=1  use_mototune_group=on  mototune_group=motohawk_vardec_path(gcb)
  motohawk_probe1 : MotoHawk_lib/Calibration & Probing Blocks/motohawk_probe  nam='RPM'  show_more=on  name_source=Use Parameter  read_level=1  view_as=Number  enum_struct={'Disabled', 'Enabled'}  vector_style=Wide Row  use_help_units=on  help=''  units=''  use_header_enum=off  row_header_enum={}  col_header_enum={}  use_precision=on  precision=''  gain=1  offset=0  exp=1  use_mototune_group=on  mototune_group=motohawk_vardec_path(gcb)
  motohawk_probe2 : MotoHawk_lib/Calibration & Probing Blocks/motohawk_probe  nam='EncoderState'  show_more=on  name_source=Use Parameter  read_level=1  view_as=Enumeration  enum_struct={'zero','ZERO_SPEED', 'POSN_UNKNOWN','ENC_SYNC_CAM_UNKNOWN','ENC_SYNC_CAM_SYNC'}  vector_style=Wide Row  use_help_units=off  help=''  units=''  use_header_enum=off  row_header_enum={}  col_header_enum={}  use_precision=off  precision=''  gain=1  offset=0  exp=1  use_mototune_group=on  mototune_group=motohawk_vardec_path(gcb)
  RPMInst : Outport
  RPM : Outport  Port=2
  wires:
  First Order Low Pass (Tunable)1/1 -> motohawk_probe1/1, RPM/1  "RPM"
  motohawk_encoder_fault/1 -> Encoder Diagnostics/1(Encoder Fault)
  motohawk_encoder_state/1 -> motohawk_probe2/1
  Data Type Conversion3/1 -> motohawk_encoder_offset/1
  Gain/1 -> Data Type Conversion3/1
  motohawk_calibration1/1 -> Gain/1
  Data Type Conversion1/1 -> motohawk_probe/1, RPMInst/1  "RPMInst"
  Data Type Conversion/1 -> First Order Low Pass (Tunable)1/1  "RPM"
  Constant/1 -> Relational Operator/1
  Relational Operator/1 -> motohawk_encoder_pseudo/1
  motohawk_calibration/1 -> Relational Operator/2, motohawk_encoder_pseudo/2
  motohawk_encoder_average_rpm/1 -> Data Type Conversion/1  "RPM"
  motohawk_encoder_instant_rpm/1 -> Data Type Conversion1/1  "RPMInst"

== system BaseEngineController_LS_128/Foreground/Inputs/LinearSensors ==
  "ACPres " : motohawk_engine_lib/Linear Sensor Characterization  SystemSampleTime=-1  nam='ACPres'  prefix='ACPres'  units='kPa Gauge'  inputunits='ADC'  parent_group=motohawk_vardec_path(gcb)  samp_time=-1
  Bus Creator3 : BusCreator  Inputs=9
  FuelOxygenationSensor : Subsystem  AncestorBlock=motohawk_engine_lib/Linear Sensor Characterization  mask(Linear Sensor Characterization){nam='FuelSens', prefix='FuelSens', units='%', inputunits='Hz', parent_group=motohawk_vardec_path(gcb), samp_time=-1}
      mask prompts: nam "Name"; units "Output Units"; inputunits "Input Units"; parent_group "MotoTune Group"; samp_time "Sample Time"
      mask help:
      | Converts from A/D Counts to Engineering Units, using a Gain and Offset.
      | Saturates the converted value around Min and Max values, and triggers a Fault when out of range.
      mask init:
      | lbl = ['Linear Sensor: ' nam ' [' units ']'];
      | group = [parent_group ' | ' nam];
      settings: RTWSystemCode=Function  RTWFcnNameOpts=Use subsystem name  RTWFileNameOpts=Use function name
      mask Display:
      | patch([0 0 1 1], [0 0.075 0.075 0], [230/255 0/255 0/255])
      | patch([0 0 1 1], [0.025 0.05 0.05 0.025], [150/255 0/255 0/255])
      | patch([0 0 1 1], [0 0.025 0.025 0], [0/255 0/255 0/255])
      | 
      | disp(lbl);
  FuelPres : motohawk_engine_lib/Linear Sensor Characterization  SystemSampleTime=-1  nam='FuelPres'  prefix='FuelPres'  units='kPa Gauge'  inputunits='ADC'  parent_group=motohawk_vardec_path(gcb)  samp_time=-1
  MAP : motohawk_engine_lib/Linear Sensor Characterization  SystemSampleTime=-1  nam='MAP'  prefix='MAP'  units='kPa'  inputunits='ADC'  parent_group=motohawk_vardec_path(gcb)  samp_time=-1
  MAPTime : motohawk_engine_lib/Linear Sensor Characterization  SystemSampleTime=-1  nam='MAPTime'  prefix='MAPTime'  units='kPa'  inputunits='ADC'  parent_group=motohawk_vardec_path(gcb)  samp_time=-1
  MAP_Crank_Synchronous : Subsystem
      mask Display: disp('Crank-Synchronous MAP');
  OilPres : motohawk_engine_lib/Linear Sensor Characterization  SystemSampleTime=-1  nam='OilPres'  prefix='OilPres'  units='psi'  inputunits='ADC'  parent_group=motohawk_vardec_path(gcb)  samp_time=-1
  SensVolts : motohawk_engine_lib/Linear Sensor Characterization  SystemSampleTime=-1  nam='SensVolt'  prefix='SensVolt'  units='Volts'  inputunits='ADC'  parent_group=motohawk_vardec_path(gcb)  samp_time=-1
  SysVolts : motohawk_engine_lib/Linear Sensor Characterization  SystemSampleTime=-1  nam='SysVolt'  prefix='SysVolt'  units='Volts'  inputunits='ADC'  parent_group=motohawk_vardec_path(gcb)  samp_time=-1
  Terminator{1..7} (7 alike) : Terminator
  motohawk_ain1 : MotoHawk_lib/Analog I//O Blocks/motohawk_ain  res_name=[]  text_resource=AN2M  code_resource=RES_ECUP  val_resource=-1  target=ECU565-128  resource_enum_str=(None)=-1,ECUP=53,DRVP=54,XDRP=55,AN1M=56,AN2M=57,AN3M=58,AN4M=59,AN5M=60,AN6M=61,AN7M=62,AN8M=63,AN9M=64,AN10M=65,AN11M=66,AN12M=67,AN13M=68,AN14M=69,AN15M=70,AN16M=71,AN17M=72,AN18M=73,AN19M=74,AN20M=75,AN21M=76,AN22M=77,AN23M=78,AN24M=79,AN25M=80,AN26M=81,AN27M=82,AN28M=83,AN29M=84,AN30M=85,AN31M=86,AN32M=87,AN33M=88,AN34M=89,O2A=90,O2B=91,XDRP_B=92,REF_14V=143  altref=5V Reference  typ=uint16  num_adc_bits=10  use_stat=off  use_vardec=on  nam='OilPresPin'  read_level=1  write_level=1  group='System | I/O Pins | Inputs Config'
  motohawk_ain14 : MotoHawk_lib/Analog I//O Blocks/motohawk_ain  res_name=[]  text_resource=DRVP  code_resource=RES_ECUP  val_resource=-1  target=ECU565-128  resource_enum_str=(None)=-1,ECUP=53,DRVP=54,XDRP=55,AN1M=56,AN2M=57,AN3M=58,AN4M=59,AN5M=60,AN6M=61,AN7M=62,AN8M=63,AN9M=64,AN10M=65,AN11M=66,AN12M=67,AN13M=68,AN14M=69,AN15M=70,AN16M=71,AN17M=72,AN18M=73,AN19M=74,AN20M=75,AN21M=76,AN22M=77,AN23M=78,AN24M=79,AN25M=80,AN26M=81,AN27M=82,AN28M=83,AN29M=84,AN30M=85,AN31M=86,AN32M=87,AN33M=88,AN34M=89,O2A=90,O2B=91,XDRP_B=92,REF_14V=143  altref=5V Reference  typ=uint16  num_adc_bits=10  use_stat=off  use_vardec=on  nam='SysVoltage'  read_level=1  write_level=1  group='System | I/O Pins | Inputs Config'
  motohawk_ain2 : MotoHawk_lib/Analog I//O Blocks/motohawk_ain  res_name=[]  text_resource=AN3M  code_resource=RES_ECUP  val_resource=-1  target=ECU565-128  resource_enum_str=(None)=-1,ECUP=53,DRVP=54,XDRP=55,AN1M=56,AN2M=57,AN3M=58,AN4M=59,AN5M=60,AN6M=61,AN7M=62,AN8M=63,AN9M=64,AN10M=65,AN11M=66,AN12M=67,AN13M=68,AN14M=69,AN15M=70,AN16M=71,AN17M=72,AN18M=73,AN19M=74,AN20M=75,AN21M=76,AN22M=77,AN23M=78,AN24M=79,AN25M=80,AN26M=81,AN27M=82,AN28M=83,AN29M=84,AN30M=85,AN31M=86,AN32M=87,AN33M=88,AN34M=89,O2A=90,O2B=91,XDRP_B=92,REF_14V=143  altref=5V Reference  typ=uint16  num_adc_bits=10  use_stat=off  use_vardec=on  nam='FuelPresPin'  read_level=1  write_level=1  group='System | I/O Pins | Inputs Config'
  motohawk_ain3 : MotoHawk_lib/Analog I//O Blocks/motohawk_ain  res_name=[]  text_resource=XDRP  code_resource=RES_ECUP  val_resource=-1  target=ECU565-128  resource_enum_str=(None)=-1,ECUP=53,DRVP=54,XDRP=55,AN1M=56,AN2M=57,AN3M=58,AN4M=59,AN5M=60,AN6M=61,AN7M=62,AN8M=63,AN9M=64,AN10M=65,AN11M=66,AN12M=67,AN13M=68,AN14M=69,AN15M=70,AN16M=71,AN17M=72,AN18M=73,AN19M=74,AN20M=75,AN21M=76,AN22M=77,AN23M=78,AN24M=79,AN25M=80,AN26M=81,AN27M=82,AN28M=83,AN29M=84,AN30M=85,AN31M=86,AN32M=87,AN33M=88,AN34M=89,O2A=90,O2B=91,XDRP_B=92,REF_14V=143  altref=5V Reference  typ=uint16  num_adc_bits=10  use_stat=off  use_vardec=on  nam='SensVoltSensorPin'  read_level=1  write_level=1  group='System | I/O Pins | Inputs Config'
  motohawk_ain4 : MotoHawk_lib/Analog I//O Blocks/motohawk_ain  res_name=[]  text_resource=AN8M  code_resource=RES_ECUP  val_resource=-1  target=ECU565-128  resource_enum_str=(None)=-1,ECUP=53,DRVP=54,XDRP=55,AN1M=56,AN2M=57,AN3M=58,AN4M=59,AN5M=60,AN6M=61,AN7M=62,AN8M=63,AN9M=64,AN10M=65,AN11M=66,AN12M=67,AN13M=68,AN14M=69,AN15M=70,AN16M=71,AN17M=72,AN18M=73,AN19M=74,AN20M=75,AN21M=76,AN22M=77,AN23M=78,AN24M=79,AN25M=80,AN26M=81,AN27M=82,AN28M=83,AN29M=84,AN30M=85,AN31M=86,AN32M=87,AN33M=88,AN34M=89,O2A=90,O2B=91,XDRP_B=92,REF_14V=143  altref=5V Reference  typ=uint16  num_adc_bits=10  use_stat=off  use_vardec=on  nam='ACPresPin'  read_level=1  write_level=1  group='System | I/O Pins | Inputs Config'
  motohawk_ain_read1 : MotoHawk_lib/Analog I//O Blocks/motohawk_ain_read  nam='MAPSensorPin'  typ=uint16
  motohawk_callout1 : motohawk_annotations_lib/motohawk_callout1  BlockType_='Mototron_harea'  desc='\fontsize{12}Read from H/W'  edit_text=Compute the mean forward body acceleration.Worry about rounding.  edit_as=255
  motohawk_callout2 : motohawk_annotations_lib/motohawk_callout1  BlockType_='Mototron_harea'  desc='\fontsize{12}Convert to Engineering Units'  edit_text=Compute the mean forward body acceleration.Worry about rounding.  edit_as=255
  motohawk_callout3 : motohawk_annotations_lib/motohawk_callout1  BlockType_='Mototron_harea'  desc='\fontsize{12}Create a Bus of Sensors'  edit_text=Compute the mean forward body acceleration.Worry about rounding.  edit_as=255
  motohawk_frequency_in : MotoHawk_lib/Advanced Digital I//O/motohawk_frequency_in  res_name=[]  text_resource=DG1M  code_resource=RES_DG1M  val_resource=-1  target=ECU565-128  resource_enum_str=(None)=-1,DG1M=93,DG2M=94,DG3M=95,DG4M=96,DG5M=102,DG6M=103,DG7M=104,SPD1=105,SPD2=106,DG8M=111  ipwm=No Duty Cycle Measurement  itrig=off  Nmax=10  edge=Rising Edge  alias=Disabled  min_freq=10  sig=Digital Input  use_vardec=on  nam='FuelSensorPin'  read_level=1  write_level=1  group='System | I/O Pins | Inputs Config'  cal_group='System | I/O Pins | Frequency In Config'
  SensorBus : Outport
  wires:
  Bus Creator3/1 -> SensorBus/1  "LinearSensors"
  motohawk_ain_read1/1 -> MAPTime/1
  MAP_Crank_Synchronous/1(ADC) -> MAP/1
  SysVolts/2 -> Terminator4/1
  SensVolts/2 -> Terminator3/1
  MAP/2 -> Terminator2/1
  MAPTime/2 -> Bus Creator3/5  "MAP_Time_Raw"
  MAPTime/1 -> Bus Creator3/4  "Map_Time"
  MAP/1 -> Bus Creator3/3  "MAP_Angular"
  SensVolts/1 -> Bus Creator3/2  "SensVolt"
  motohawk_ain3/1 -> SensVolts/1
  SysVolts/1 -> Bus Creator3/1  "SysVolt"
  motohawk_ain14/1 -> SysVolts/1
  motohawk_ain1/1 -> OilPres/1
  OilPres/2 -> Terminator1/1
  OilPres/1 -> Bus Creator3/6  "OilPres"
  motohawk_frequency_in/1 -> FuelOxygenationSensor/1(ADC)
  FuelOxygenationSensor/2(EngUnitsRaw) -> Terminator6/1
  motohawk_ain2/1 -> FuelPres/1
  FuelPres/2 -> Terminator7/1
  FuelOxygenationSensor/1(EngUnitsFilt) -> Bus Creator3/7  "FuelSense"
  FuelPres/1 -> Bus Creator3/8  "FuelPres"
  motohawk_ain4/1 -> "ACPres "/1
  "ACPres "/1 -> Bus Creator3/9  "ACPres"
  "ACPres "/2 -> Terminator5/1

== system BaseEngineController_LS_128/Foreground/Inputs/NonLinearSensors ==
  Bus Creator1 : BusCreator  Inputs=10
  Fuel Level : Subsystem  TreatAsAtomicUnit=on
  Temp Sensors : Subsystem  TreatAsAtomicUnit=on
  motohawk_trigger : MotoHawk_lib/Trigger Blocks/motohawk_trigger  Tag=Trigger  trigger=FGND_5XRTI_PERIODIC  function_name=Trigger_FGND_5XRTI_PERIODIC_9815p0006  priority_order=1  inherited=on  run_disabled=off  override_app_monitor=off  target=ECU565_128
  motohawk_trigger1 : MotoHawk_lib/Trigger Blocks/motohawk_trigger  Tag=Trigger  trigger=FGND_5XRTI_PERIODIC  function_name=Trigger_FGND_5XRTI_PERIODIC_9816p0004  priority_order=1  inherited=on  run_disabled=off  override_app_monitor=off  target=ECU565_128
  SensorBus : Outport
  wires:
  Bus Creator1/1 -> SensorBus/1  "NonLinearSensors"
  Temp Sensors/2(ECT_Raw) -> Bus Creator1/2  "ECT_Raw"
  Temp Sensors/4(IAT_Raw) -> Bus Creator1/4  "IAT_Raw"
  Temp Sensors/3(IAT) -> Bus Creator1/3  "IAT"
  Temp Sensors/1(ECT) -> Bus Creator1/1  "ECT"
  motohawk_trigger/1 -> Temp Sensors/Trigger
  Temp Sensors/5(EVAP) -> Bus Creator1/5  "EVAP"
  Temp Sensors/6(EVAP_Raw) -> Bus Creator1/6  "EVAP_Raw"
  Temp Sensors/8(CAT_Raw) -> Bus Creator1/8  "CAT_Raw"
  Temp Sensors/7(CAT) -> Bus Creator1/7  "CAT"
  Fuel Level/1(Fuel Lvl) -> Bus Creator1/9  "Fuel_Lvl"
  Fuel Level/2(Fuel Lvl Raw) -> Bus Creator1/10  "Fuel_Lvl_Raw"
  motohawk_trigger1/1 -> Fuel Level/Trigger
